simulink model "RightArmAgent"  (Simulink 6.2)
settings: Solver=ode45  SolverMode=SingleTasking  StartTime=0.0  StopTime=10.0  RelTol=1e-3  AbsTol=1e-6
settings Model: Creator=The MathWorks Inc.  LastModifiedBy=suarezjl  ExtModeTrigMode=oneshot  ExtModeArmWhenConnect=off  ExtModeAutoUpdateStatusClock=off
settings DataIOCC: LimitDataPoints=off  SignalLoggingName=logsOut
settings OptimizationCC: BooleanDataType=off  InlineInvariantSignals=on
settings DebuggingCC: CheckExecutionContextPreStartOutputMsg=on  CheckExecutionContextRuntimeOutputMsg=on  IntegerOverflowMsg=none
settings HardwareCC: TargetUnknown=on
settings ModelReferenceCC: UpdateModelReferenceTargets=IfOutOfDate

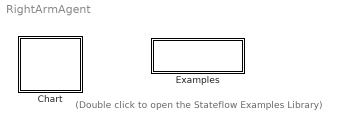
== system RightArmAgent ==
  note: (Double click to open the
      | Stateflow Examples Library)
  Chart : Stateflow chart
  Examples : Subsystem
      settings: OpenFcn=sf('Private','sf_examples')
      mask Display: disp('Examples')

== system RightArmAgent/Examples ==

== stateflow chart Chart ==
  state InitialArmRoutine
    Popeye\RightReachDemo\RightArm\HomingController.ComputeHomingPressures()
    Popeye\RightReachDemo\RightArm\SampleIndPressure.HW_IO_6()
    Popeye\RightReachDemo\RightArm\StateMachine.Wait(50)
  state InitializeFunctions
    Popeye\RightReachDemo\RightArm\HomingController.Initial()
    Popeye\RightReachDemo\RightArm\SampleIndPressure.Initialize()
    Popeye\RightReachDemo\RightArm\PIDNonLinCtrl.Initial()
    Popeye\RightReachDemo\RightArm\ForwardKinematics.Initialize()
    Popeye\RightReachDemo\RightArm\InverseKinematics.Initialize()
    Popeye\RightReachDemo\RightArm\SampleIndPressure.Disable_ZMasking()
  state WriteHomeDesiredLogicalAngles
    Popeye\RightReachDemo\RightArm\SampleIndPressure.Enable_ZMasking()
    Popeye\RightReachDemo\RightArm\SampleIndPressure.WriteHomePositions()
  state LoadHomePosition
    Popeye\RightReachDemo\RightArm\SampleIndPressure.HW_IO_6()
    Popeye\RightReachDemo\RightArm\PIDNonLinCtrl.PID_NonLin_6Press()
    Popeye\RightReachDemo\RightArm\ForwardKinematics.ForwardKinematics()
    Popeye\RightReachDemo\RightArm\InverseKinematics.InverseKinematics()
  state PID_NonLinCtrlLoop
    Popeye\RightReachDemo\RightArm\Filter.FilterDesiredAngles()
    Popeye\RightReachDemo\RightArm\PIDNonLinCtrl.PID_NonLin_12Press()
    Popeye\RightReachDemo\RightArm\SampleIndPressure.HW_IO_12()
    Popeye\RightReachDemo\RightArm\PIDNonLinCtrl.Read_CurrentPressure()
    Popeye\RightReachDemo\RightArm\ForwardKinematics.ForwardKinematics()
    Popeye\RightReachDemo\RightArm\InverseKinematics.InverseKinematics()
    Popeye\RightReachDemo\RightArm\StateMachine.Wait(50)
  (default) -> InitializeFunctions : Start
  InitialArmRoutine -> InitialArmRoutine [order 1] : Default
  InitializeFunctions -> InitialArmRoutine : Always
  WriteHomeDesiredLogicalAngles -> LoadHomePosition : Always
  LoadHomePosition -> PID_NonLinCtrlLoop : Always
  InitialArmRoutine -> WriteHomeDesiredLogicalAngles [order 2] : Signal="Go to next state"
  PID_NonLinCtrlLoop -> PID_NonLinCtrlLoop : Default
